simulink model "gm_dvfs_zed_simple_interface"  (R2025b)
settings: Solver=FixedStepDiscrete  StartTime=0.0  StopTime=10.0  FixedStep=0.1  RelTol=1e-3  EnableMultiTasking=on
undefined symbols (not defined in the file or in its folder): AXI4, Lite
libraries: axiinterfacelib x3, hdlsllib x3
settings Model: Creator=Vimal Rency  LastModifiedBy=Vimal Rency
settings SolverCC: ConcurrentTasks=on  PositivePriorityOrder=on
settings OptimizationCC: BlockReduction=off  ConditionallyExecuteInputs=off  EnhancedBackFolding=on  PassReuseOutputArgsAs=Individual arguments  ZeroExternalMemoryAtStartup=off  ZeroInternalMemoryAtStartup=off  MaxStackSize=64  OptimizeBlockOrder=speed  DifferentSizesBufferReuse=on  OptimizationCustomize=off  EfficientTunableParamExpr=on
settings DebuggingCC: ParameterTunabilityLossMsg=error
settings HardwareCC: ProdBitPerPointer=32.0  ProdBitPerSizeT=32.0  ProdBitPerPtrDiffT=32.0  ProdLargestAtomicInteger=Long  ProdLargestAtomicFloat=Double  ProdWordSize=32.0  ProdLongLongMode=on  ProdHWDeviceType=ARM Compatible->ARM Cortex-A (32-bit)  TargetBitPerPointer=64.0  TargetBitPerSizeT=64.0  TargetBitPerPtrDiffT=64.0  TargetLongLongMode=on  TargetIntDivRoundTo=Zero  TargetEndianess=LittleEndian  TargetWordSize=64.0  TargetHWDeviceType=Custom Processor->MATLAB Host Computer
settings ModelReferenceCC: ModelReferenceNumInstancesAllowed=Single
settings SFSimCC: MATLABDynamicMemAlloc=off
settings RTWCC: SystemTargetFile=ert.tlc  HardwareBoard=ZedBoard  TLCOptions="-aInlineSetEventsForThisBaseRateFcn=TLC_FALSE -aSuppressMultiTaskScheduler=TLC_FALSE  -aRateBasedStepFcn=0"  TemplateMakefile=ert_default_tmf  Toolchain=Linaro AArch32 Linux v6.3.1  Description=Embedded Coder
settings CodeAppCC: ForceParamTrailComments=on  IgnoreCustomStorageClasses=off  OperatorAnnotations=on  SimulinkDataObjDesc=on  SFDataObjDesc=on  InsertBlockDesc=on
settings ERTTargetCC: InlinedParameterPlacement=Hierarchical  SubcomponentCodeInterfacePackaging=Nonreusable function

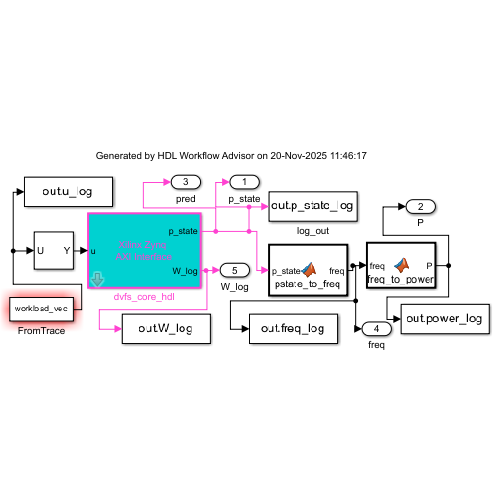
[thumbnail: Simulink's stored preview of the top-level diagram]
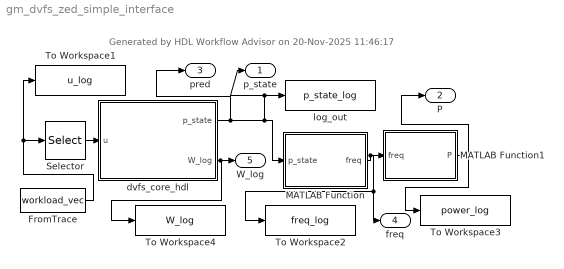
== system gm_dvfs_zed_simple_interface ==
  note: Generated by HDL Workflow Advisor on 20-Nov-2025 11:46:17
  FromTrace : FromWorkspace  VariableName=workload_vec
  MATLAB Function : MATLAB Function  TreatAsAtomicUnit=on
  MATLAB Function1 : MATLAB Function  TreatAsAtomicUnit=on
  Selector : Selector  NumberOfDimensions=2  InputPortWidth=3  IndexOptions=Select all,Index vector (dialog)  Indices=[1 3],1  OutputSizes=1,1
  To Workspace1 : ToWorkspace  VariableName=u_log  SampleTime=-1
  To Workspace2 : ToWorkspace  VariableName=freq_log  SampleTime=-1
  To Workspace3 : ToWorkspace  VariableName=power_log  SampleTime=-1
  To Workspace4 : ToWorkspace  VariableName=W_log  SampleTime=-1
  dvfs_core_hdl : Subsystem  TreatAsAtomicUnit=on  mask(AXI4-Lite/AXI4 Interface){}
      mask help:
      | This is an automatically generated subsystem block.
      | This contains the AXI interface blocks that communicate with the dvfs_core_ip IPCore generated from dvfs_zed_simple/dvfs_core_hdl subsystem.
      mask Display: disp(sprintf('Xilinx Zynq \nAXI Interface'));
  log_out : ToWorkspace  VariableName=p_state_log  SampleTime=-1
  p_state : Outport
  P : Outport  Port=2
  pred : Outport  Port=3
  freq : Outport  Port=4
  W_log : Outport  Port=5
  wires:
  Selector/1 -> dvfs_core_hdl/1(u)
  dvfs_core_hdl/1(p_state) -> p_state/1, log_out/1, MATLAB Function/1(p_state), pred/1
  dvfs_core_hdl/2(W_log) -> To Workspace4/1, W_log/1
  MATLAB Function/1(freq) -> freq/1, To Workspace2/1, MATLAB Function1/1(freq)
  MATLAB Function1/1(P) -> To Workspace3/1, P/1
  FromTrace/1 -> To Workspace1/1, Selector/1

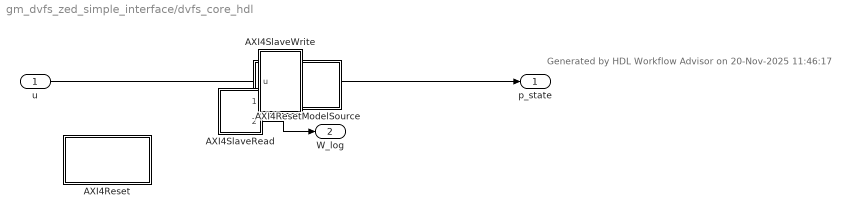
== system gm_dvfs_zed_simple_interface/dvfs_core_hdl ==
  note: Generated by HDL Workflow Advisor on 20-Nov-2025 11:46:17
  u : Inport
  AXI4Reset : Subsystem  mask(System Start){ShowInLibBrowser=0}
      mask prompts: ShowInLibBrowser "Simulink:masks:CustCodeMaskParam1_MP"
      settings: CopyFcn=cccopyfcn(gcb)  OpenFcn=ccopenfcn('System Start Function')
      mask Help: eval('feval(''rtwprivate'',''rtwhelpview'',''rtw_sys_start_block'')');
      mask Display: disp('System\nStart');
  AXI4ResetModelSource : Subsystem  mask(Model Source){ShowInLibBrowser=0}
      mask prompts: ShowInLibBrowser "Simulink:masks:CustCodeMaskParam1_MP"
      settings: CopyFcn=cccopyfcn(gcb)  OpenFcn=ccopenfcn('Model Source')
      mask Help: eval('feval(''rtwprivate'',''rtwhelpview'',''rtw_model_source_block'')');
      mask Display: disp('Model\nSource');
  AXI4SlaveRead : Subsystem  Priority=10
  AXI4SlaveWrite : Subsystem  Priority=1
  p_state : Outport
  W_log : Outport  Port=2
  wires:
  u/1 -> AXI4SlaveWrite/1(u)
  AXI4SlaveRead/1(p_state) -> p_state/1
  AXI4SlaveRead/2(W_log) -> W_log/1

== system gm_dvfs_zed_simple_interface/dvfs_core_hdl/AXI4Reset ==

== system gm_dvfs_zed_simple_interface/dvfs_core_hdl/AXI4ResetModelSource ==

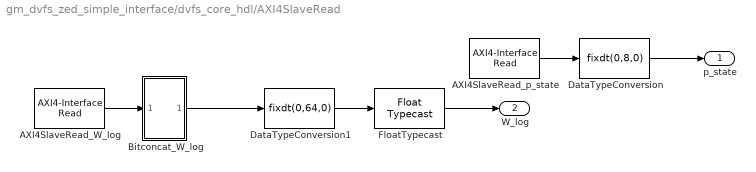
== system gm_dvfs_zed_simple_interface/dvfs_core_hdl/AXI4SlaveRead ==
  AXI4SlaveRead_W_log : axiinterfacelib/AXI4-Interface Read  Priority=4  AXIInterfaceType=AXI4-Lite  DeviceName=/dev/mwipcore  RegisterOffset=hex2dec('110')  DataLength=2  DataType=uint32  SampleTime=-1  blockPlatform=ZYNQ  SimulateUsing=Interpreted Execution
  AXI4SlaveRead_p_state : axiinterfacelib/AXI4-Interface Read  Priority=3  AXIInterfaceType=AXI4-Lite  DeviceName=/dev/mwipcore  RegisterOffset=hex2dec('10C')  DataLength=1  DataType=uint32  SampleTime=-1  blockPlatform=ZYNQ  SimulateUsing=Interpreted Execution
  Bitconcat_W_log : Subsystem
  DataTypeConversion : DataTypeConversion  OutDataTypeStr=fixdt(0,8,0)  ConvertRealWorld=Stored Integer (SI)  SaturateOnIntegerOverflow=off  RndMeth=Floor
  DataTypeConversion1 : DataTypeConversion  OutDataTypeStr=fixdt(0,64,0)  ConvertRealWorld=Stored Integer (SI)  SaturateOnIntegerOverflow=off  RndMeth=Floor
  FloatTypecast : FloatTypecast
  p_state : Outport
  W_log : Outport  Port=2
  wires:
  AXI4SlaveRead_W_log/1 -> Bitconcat_W_log/1(In1)
  DataTypeConversion/1 -> p_state/1
  FloatTypecast/1 -> W_log/1
  DataTypeConversion1/1 -> FloatTypecast/1
  AXI4SlaveRead_p_state/1 -> DataTypeConversion/1
  Bitconcat_W_log/1(Out1) -> DataTypeConversion1/1

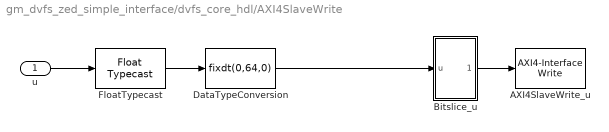
== system gm_dvfs_zed_simple_interface/dvfs_core_hdl/AXI4SlaveWrite ==
  u : Inport
  AXI4SlaveWrite_u : axiinterfacelib/AXI4-Interface Write  Priority=2  AXIInterfaceType=AXI4-Lite  DeviceName=/dev/mwipcore  RegisterOffset=hex2dec('100')  blockPlatform=ZYNQ  SimulateUsing=Interpreted execution
  Bitslice_u : Subsystem
  DataTypeConversion : DataTypeConversion  OutDataTypeStr=fixdt(0,64,0)  ConvertRealWorld=Stored Integer (SI)  SaturateOnIntegerOverflow=off  RndMeth=Floor
  FloatTypecast : FloatTypecast
  wires:
  Bitslice_u/1(Out1) -> AXI4SlaveWrite_u/1
  DataTypeConversion/1 -> Bitslice_u/1(u)
  u/1 -> FloatTypecast/1
  FloatTypecast/1 -> DataTypeConversion/1

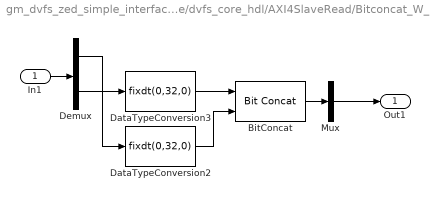
== system gm_dvfs_zed_simple_interface/dvfs_core_hdl/AXI4SlaveRead/Bitconcat_W_log ==
  In1 : Inport
  BitConcat : hdlsllib/Logic and Bit Operations/Bit Concat  numInputs=2
  DataTypeConversion2 : DataTypeConversion  OutDataTypeStr=fixdt(0,32,0)  ConvertRealWorld=Stored Integer (SI)  SaturateOnIntegerOverflow=off  RndMeth=Floor
  DataTypeConversion3 : DataTypeConversion  OutDataTypeStr=fixdt(0,32,0)  ConvertRealWorld=Stored Integer (SI)  SaturateOnIntegerOverflow=off  RndMeth=Floor
  Demux : Demux  Outputs=2
  Mux : Mux  Inputs=1
  Out1 : Outport
  wires:
  Mux/1 -> Out1/1
  In1/1 -> Demux/1
  Demux/2 -> DataTypeConversion3/1
  Demux/1 -> DataTypeConversion2/1
  DataTypeConversion3/1 -> BitConcat/1
  DataTypeConversion2/1 -> BitConcat/2
  BitConcat/1 -> Mux/1

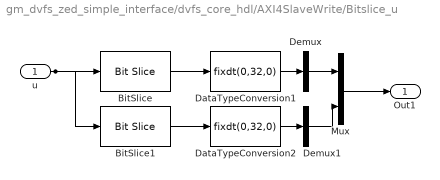
== system gm_dvfs_zed_simple_interface/dvfs_core_hdl/AXI4SlaveWrite/Bitslice_u ==
  u : Inport
  BitSlice : hdlsllib/Logic and Bit Operations/Bit Slice  lidx=31  ridx=0
  BitSlice1 : hdlsllib/Logic and Bit Operations/Bit Slice  lidx=63  ridx=32
  DataTypeConversion1 : DataTypeConversion  OutDataTypeStr=fixdt(0,32,0)  ConvertRealWorld=Stored Integer (SI)  SaturateOnIntegerOverflow=off  RndMeth=Floor
  DataTypeConversion2 : DataTypeConversion  OutDataTypeStr=fixdt(0,32,0)  ConvertRealWorld=Stored Integer (SI)  SaturateOnIntegerOverflow=off  RndMeth=Floor
  Demux : Demux  Outputs=1
  Demux1 : Demux  Outputs=1
  Mux : Mux  Inputs=2
  Out1 : Outport
  wires:
  BitSlice/1 -> DataTypeConversion1/1
  u/1 -> BitSlice1/1, BitSlice/1
  Mux/1 -> Out1/1
  BitSlice1/1 -> DataTypeConversion2/1
  DataTypeConversion1/1 -> Demux/1
  DataTypeConversion2/1 -> Demux1/1
  Demux/1 -> Mux/1
  Demux1/1 -> Mux/2

== matlab function gm_dvfs_zed_simple_interface/MATLAB Function1 ==
  data: freq input; P output
function P = freq_to_power(freq)

% simple model: Power ∝ frequency
P = 0.01 * freq;   % scale as you want (mW)

end

== matlab function gm_dvfs_zed_simple_interface/MATLAB Function ==
  data: p_state input; freq output
function freq = pstate_to_freq(p_state)

switch p_state
    case 0
        freq = 100;   % MHz
    case 1
        freq = 200;
    case 2
        freq = 300;
    otherwise
        freq = 0;
end

end
